simulink model "obtencion_datos_ESP32"  (R2023b)
settings: Solver=ode4  StartTime=0.0  StopTime=20.0  FixedStep=0.001  RelTol=1e-3
undefined symbols (not defined in the file or in its folder): LF
libraries: instrumentseriallib x3
settings Model: Creator=saulc  LastModifiedBy=saulc

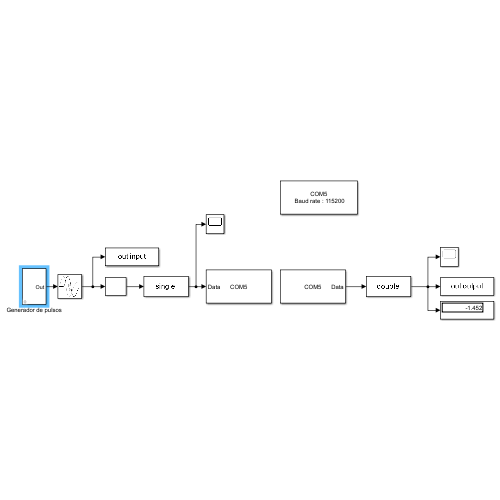
[thumbnail: Simulink's stored preview of the top-level diagram]
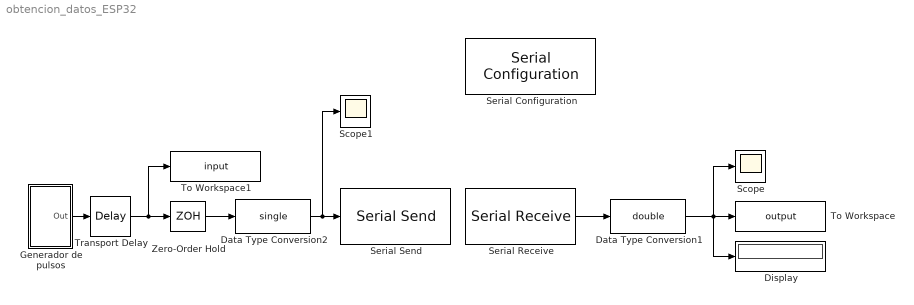
== system obtencion_datos_ESP32 ==
  Data Type Conversion1 : DataTypeConversion  OutDataTypeStr=double  SaturateOnIntegerOverflow=off  RndMeth=Floor
  Data Type Conversion2 : DataTypeConversion  OutDataTypeStr=single  SaturateOnIntegerOverflow=off  RndMeth=Floor
  Display : Display
  Generador de pulsos : Subsystem  mask{A=20, P=8}
      mask prompts: A "Amplitud"; P "Periodo"
  Scope : Scope
  Scope1 : Scope
  Serial Configuration : instrumentseriallib/Serial Configuration  Priority=-200000  PortSel=COM5  Port=COM5  ComPort=COM5  BaudRate=115200  DataBits=8  Parity=none  StopBits=1  ByteOrder=little-endian  FlowControl=none  Timeout=10  SimulateUsing=Interpreted execution  BlockInModel=on  aMode=1
      settings: LibrarySourceBlock=c2000lib/Host Communication/Serial Configuration
  Serial Receive : instrumentseriallib/Serial Receive  Priority=1  PortSel=COM5  Port=COM5  ComPort=COM5  DataType=single  SaveDataType=uint8  ToggleHeader=on  Header='V'  ToggleTerminator=on  Terminator=LF ('\n')  CustomTerminator=[]  InputFormat=Column major  ToggleDataSize=on  DataSize=[1 1]  EnableBlockingMode=on  ActionDataUnavailable=Output custom value  ActionWhenDataUnavailable=Output custom value  CustomValue=0  SampleTime=0.02  SimulateUsing=Interpreted execution  BlockInModel=on  aMode=1
      settings: LibrarySourceBlock=embeddedtargetslib/Host Communication/Serial Receive
  Serial Send : instrumentseriallib/Serial Send  Priority=1  PortSel=COM5  Port=COM5  ComPort=COM5  Header=[]  Terminator=<none>  CustomTerminator=[]  EnableBlockingMode=on  SimulateUsing=Interpreted execution  BlockInModel=on  aMode=1
      settings: LibrarySourceBlock=embeddedtargetslib/Host Communication/Serial Send
  To Workspace : ToWorkspace  VariableName=output  SampleTime=0.001
      settings: Save2DSignal=2-D array (concatenate along first dimension)
  To Workspace1 : ToWorkspace  VariableName=input  SampleTime=0.001
      settings: Save2DSignal=2-D array (concatenate along first dimension)
  Transport Delay : TransportDelay  DelayTime=2
  Zero-Order Hold : ZeroOrderHold  SampleTime=0.05
  wires:
  Serial Receive/1 -> Data Type Conversion1/1
  Data Type Conversion1/1 -> To Workspace/1, Display/1, Scope/1
  Generador de pulsos/1(Out) -> Transport Delay/1
  Zero-Order Hold/1 -> Data Type Conversion2/1
  Data Type Conversion2/1 -> Scope1/1, Serial Send/1
  Transport Delay/1 -> To Workspace1/1, Zero-Order Hold/1

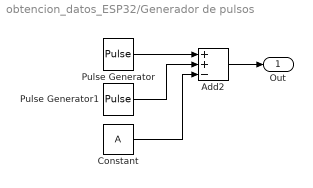
== system obtencion_datos_ESP32/Generador de pulsos ==
  Add2 : Sum  Inputs=++-
  Constant : Constant  Value=A
  Pulse Generator : DiscretePulseGenerator  PulseType=Time based  Amplitude=A  Period=P  PulseWidth=50
  Pulse Generator1 : DiscretePulseGenerator  PulseType=Time based  Amplitude=A  Period=P  PulseWidth=50  PhaseDelay=P/4
  Out : Outport
  wires:
  Pulse Generator1/1 -> Add2/2
  Constant/1 -> Add2/3
  Pulse Generator/1 -> Add2/1
  Add2/1 -> Out/1
